simulink model "Sim_Riementrieb"  (Simulink 8.0)
settings: Solver=ode45  StartTime=0.0  StopTime=3.5  MaxStep=1e-3  RelTol=1e-7  AbsTol=1e-7
InitFcn:
  | set_parameter
undefined symbols (not defined in the file or in its folder): mitRegler
libraries: cstblocks x4
settings Model: Creator=wke  LastModifiedBy=cds-lue-1
settings SolverCC: ShapePreserveControl=EnableAll
settings DataIOCC: SignalLoggingSaveFormat=ModelDataLogs
settings DebuggingCC: FcnCallInpInsideContextMsg=UseLocalSettings  StrictBusMsg=Warning
settings SFSimCC: SimParseCustomCode=off
settings CodeAppCC: CustomSymbolStrType=$N$R$M_T  InternalIdentifier=Shortened
settings GRTTargetCC: CombineOutputUpdateFcns=off  GRTInterface=on

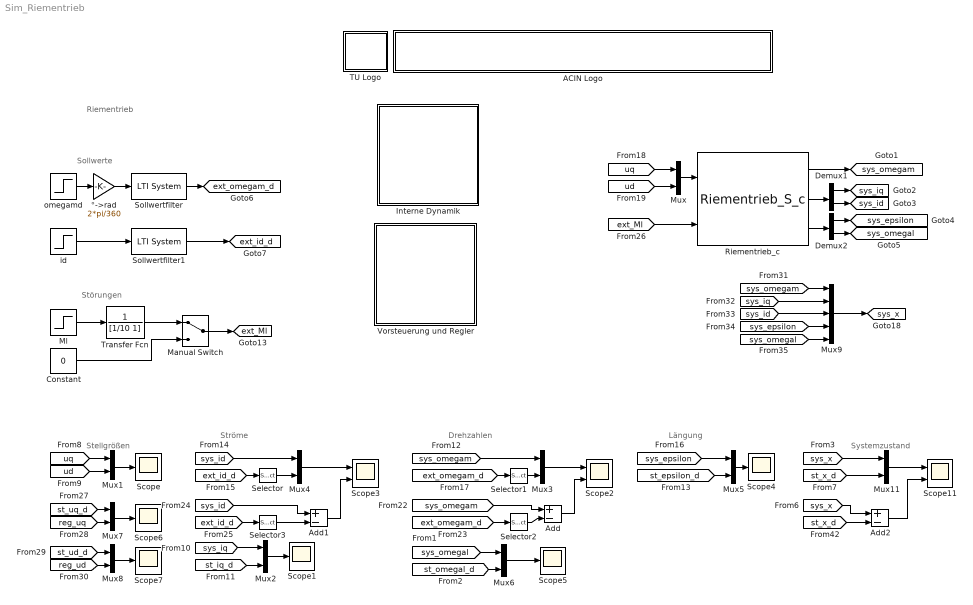
== system Sim_Riementrieb ==
  note: Riementrieb
  note: Sollwerte
  note: Stellgrößen
  note: Ströme
  note: Drehzahlen
  note: Längung
  note: Störungen
  note: Systemzustand
  ACIN Logo : Subsystem
      mask init:
      | s = get_param(gcb,'UserData');
      mask Display:
      | image(s.logo,[0 0 439 45]);
      | %axis image
  Add : Sum  Inputs=+-
  Add1 : Sum  Inputs=+-
  Add2 : Sum  Inputs=+-
  Constant : Constant  Value=0
  Demux1 : Demux  Outputs=2
  Demux2 : Demux  Outputs=2
  Interne Dynamik : Subsystem
  Manual Switch : ManualSwitch
  Ml : Step  Time=2.5  After=0.1  SampleTime=0
  Mux{,1..8,11} (10 alike) : Mux  Inputs=2
  Mux9 : Mux  Inputs=5
  Riementrieb_c : S-Function  FunctionName=Riementrieb_S_c  Parameters=parSys  EnableBusSupport=off
      mask Display:
      | port_label('input',1,'uq,ud');
      | port_label('input',2,'Ml');
      | port_label('output',1,'omegam');
      | port_label('output',2,'iq,id');
      | port_label('output',3,'epsilon,omegal');
  Scope{,1,4..7} (6 alike) : Scope
      Scope settings: YMin=-1  YMax=1
      Scope1 settings: YMin=-300000  YMax=275000
      Scope4 settings: YMin=-0.008  YMax=0.008  SaveName=ScopeData4
      Scope5 settings: YMin=0  YMax=7  SaveName=ScopeData5
      Scope6 settings: YMin=-1.66533e-016  YMax=2.4  SaveName=ScopeData6
      Scope7 settings: YMin=-1.66533e-016  YMax=2.4  SaveName=ScopeData7
  Scope11 : Scope  NumInputPorts=2
      settings: YMin=-300000~-5  YMax=275000~5  SaveName=ScopeData11
  Scope2 : Scope  NumInputPorts=2
      settings: TimeRange=0.3051681706316654  YMin=104.717~-0.0031225  YMax=104.72~-0.00282512  SaveName=ScopeData2
  Scope3 : Scope  NumInputPorts=2
      settings: TimeRange=1.762100082034454  YMin=0.00508121~-5  YMax=0.107262~5  SaveName=ScopeData3
  Selector : Selector  InputPortWidth=2  IndexOptions=Index vector (dialog)  Indices=[1]  OutputSizes=1
  Selector1 : Selector  InputPortWidth=3  IndexOptions=Index vector (dialog)  Indices=[1]  OutputSizes=1
  Selector2 : Selector  InputPortWidth=3  IndexOptions=Index vector (dialog)  Indices=[1]  OutputSizes=1
  Selector3 : Selector  InputPortWidth=2  IndexOptions=Index vector (dialog)  Indices=[1]  OutputSizes=1
  Sollwertfilter : cstblocks/LTI System  sys=parReg.ssSF  IC=[]
  Sollwertfilter1 : cstblocks/LTI System  sys=parReg.ssSFi  IC=[]
  TU Logo : Subsystem
      mask init:
      | s = get_param(gcb,'UserData');
      mask Display: image(s.logo,[0 0 45 45]);
  Transfer Fcn : TransferFcn  Denominator=[1/10 1]
  Vorsteuerung und Regler : Subsystem
  id : Step  Time=0.5  After=0.1  SampleTime=0
  omegamd : Step  Time=1.5  After=1000/60*360  SampleTime=0
  °->rad : Gain  Gain=2*pi/360
  tag scope: ext_Ml=global, ext_id_d=global, ext_omegam_d=global, sys_epsilon=global, sys_id=global, sys_iq=global, sys_omegal=global, sys_omegam=global, sys_x=global
  wires:
  Mux/1 -> Riementrieb_c/1
  °->rad/1 -> Sollwertfilter/1
  Sollwertfilter/1 -> [ext_omegam_d]
  Demux1/1 -> [sys_iq]
  Demux1/2 -> [sys_id]
  Demux2/1 -> [sys_epsilon]
  Demux2/2 -> [sys_omegal]
  Sollwertfilter1/1 -> [ext_id_d]
  id/1 -> Sollwertfilter1/1
  [uq] -> Mux1/1
  [ud] -> Mux1/2
  Mux1/1 -> Scope/1
  [sys_iq] -> Mux2/1
  [st_iq_d] -> Mux2/2
  Mux2/1 -> Scope1/1
  [sys_omegam] -> Mux3/1
  Mux3/1 -> Scope2/1
  [sys_id] -> Mux4/1
  [ext_id_d] -> Selector/1
  Mux4/1 -> Scope3/1
  [sys_epsilon] -> Mux5/1
  Mux5/1 -> Scope4/1
  [sys_omegal] -> Mux6/1
  Mux6/1 -> Scope5/1
  [ext_omegam_d] -> Selector1/1
  Selector1/1 -> Mux3/2
  Selector/1 -> Mux4/2
  [st_epsilon_d] -> Mux5/2
  [st_omegal_d] -> Mux6/2
  Add/1 -> Scope2/2
  [sys_omegam] -> Add/1
  [ext_omegam_d] -> Selector2/1
  Selector2/1 -> Add/2
  Add1/1 -> Scope3/2
  [sys_id] -> Add1/1
  [ext_id_d] -> Selector3/1
  Selector3/1 -> Add1/2
  Ml/1 -> Transfer Fcn/1
  omegamd/1 -> °->rad/1
  [ext_Ml] -> Riementrieb_c/2
  [st_uq_d] -> Mux7/1
  [reg_uq] -> Mux7/2
  Mux7/1 -> Scope6/1
  [st_ud_d] -> Mux8/1
  [reg_ud] -> Mux8/2
  Mux8/1 -> Scope7/1
  Riementrieb_c/2 -> Demux1/1
  Riementrieb_c/3 -> Demux2/1
  Riementrieb_c/1 -> [sys_omegam]
  [sys_omegam] -> Mux9/1
  [sys_iq] -> Mux9/2
  [sys_id] -> Mux9/3
  [sys_epsilon] -> Mux9/4
  [sys_omegal] -> Mux9/5
  Mux9/1 -> [sys_x]
  Mux11/1 -> Scope11/1
  [sys_x] -> Mux11/1
  [st_x_d] -> Mux11/2
  [uq] -> Mux/1
  [ud] -> Mux/2
  Add2/1 -> Scope11/2
  [sys_x] -> Add2/1
  [st_x_d] -> Add2/2
  Transfer Fcn/1 -> Manual Switch/1
  Constant/1 -> Manual Switch/2
  Manual Switch/1 -> [ext_Ml]

== system Sim_Riementrieb/ACIN Logo ==

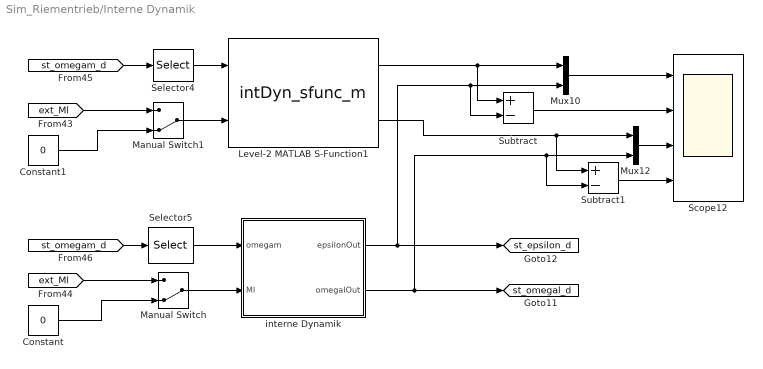
== system Sim_Riementrieb/Interne Dynamik ==
  Constant : Constant  Value=0
  Constant1 : Constant  Value=0
  Level-2 MATLAB S-Function1 : M-S-Function  FunctionName=intDyn_sfunc_m  Parameters=parIndDyn
  Manual Switch : ManualSwitch  CurrentSetting=0
  Manual Switch1 : ManualSwitch  CurrentSetting=0
  Mux10 : Mux  Inputs=2
  Mux12 : Mux  Inputs=2
  Scope12 : Scope  NumInputPorts=4
      settings: YMin=-5~-5~-5~-5  YMax=5~5~5~5  SaveName=ScopeData12
  Selector4 : Selector  InputPortWidth=3  IndexOptions=Index vector (dialog)  Indices=[1]  OutputSizes=1
  Selector5 : Selector  InputPortWidth=3  IndexOptions=Index vector (dialog)  Indices=[1]  OutputSizes=1
  Subtract : Sum  Inputs=+-
  Subtract1 : Sum  Inputs=+-
  interne Dynamik : MATLAB Function  TreatAsAtomicUnit=on
  tag scope: st_epsilon_d=global, st_omegal_d=global
  wires:
  Mux12/1 -> Scope12/3
  Level-2 MATLAB S-Function1/1 -> Mux10/1, Subtract/1
  Subtract1/1 -> Scope12/4
  interne Dynamik/1(epsilonOut) -> Mux10/2, Subtract/2, [st_epsilon_d]
  Subtract/1 -> Scope12/2
  interne Dynamik/2(omegalOut) -> Subtract1/2, Mux12/2, [st_omegal_d]
  [st_omegam_d] -> Selector4/1
  Selector4/1 -> Level-2 MATLAB S-Function1/1
  Level-2 MATLAB S-Function1/2 -> Subtract1/1, Mux12/1
  Mux10/1 -> Scope12/1
  Selector5/1 -> interne Dynamik/1(omegam)
  [st_omegam_d] -> Selector5/1
  Manual Switch/1 -> interne Dynamik/2(Ml)
  [ext_Ml] -> Manual Switch/1
  Constant/1 -> Manual Switch/2
  Manual Switch1/1 -> Level-2 MATLAB S-Function1/2
  [ext_Ml] -> Manual Switch1/1
  Constant1/1 -> Manual Switch1/2

== system Sim_Riementrieb/TU Logo ==

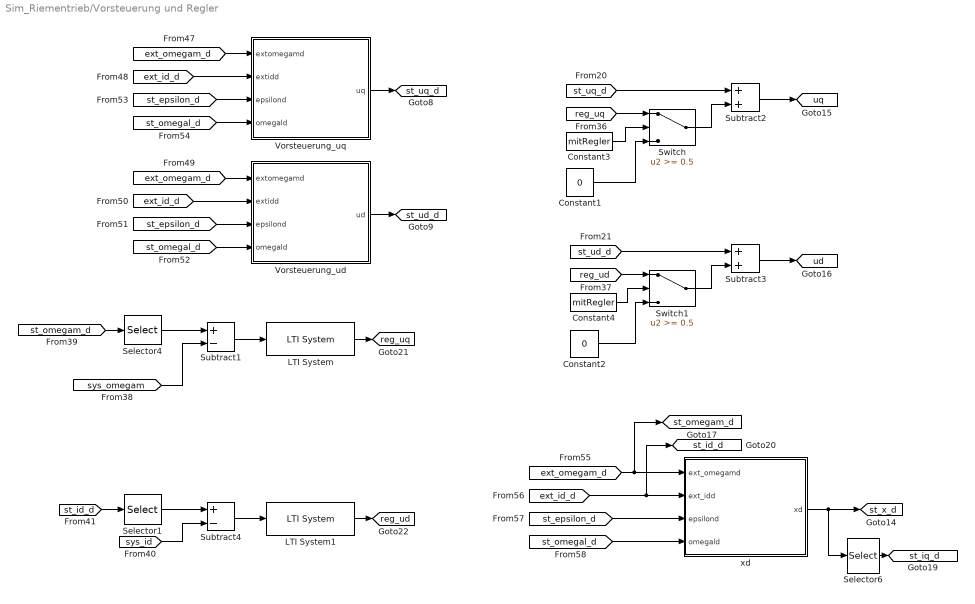
== system Sim_Riementrieb/Vorsteuerung und Regler ==
  Constant1 : Constant  Value=0
  Constant2 : Constant  Value=0
  Constant3 : Constant  Value=mitRegler
  Constant4 : Constant  Value=mitRegler
  LTI System : cstblocks/LTI System  sys=Rz_uq  IC=[]
  LTI System1 : cstblocks/LTI System  sys=Rz_ud  IC=[]
  Selector1 : Selector  InputPortWidth=2  IndexOptions=Index vector (dialog)  Indices=[1]  OutputSizes=1
  Selector4 : Selector  InputPortWidth=3  IndexOptions=Index vector (dialog)  Indices=[1]  OutputSizes=1
  Selector6 : Selector  InputPortWidth=5  IndexOptions=Index vector (dialog)  Indices=[2]  OutputSizes=1
  Subtract1 : Sum  Inputs=+-
  Subtract2 : Sum
  Subtract3 : Sum
  Subtract4 : Sum  Inputs=+-
  Switch : Switch  Threshold=0.5
  Switch1 : Switch  Threshold=0.5
  Vorsteuerung_ud : MATLAB Function  TreatAsAtomicUnit=on
  Vorsteuerung_uq : MATLAB Function  TreatAsAtomicUnit=on
  xd : MATLAB Function  TreatAsAtomicUnit=on
  tag scope: reg_ud=global, reg_uq=global, st_id_d=global, st_iq_d=global, st_omegam_d=global, st_ud_d=global, st_uq_d=global, st_x_d=global, ud=global, uq=global
  wires:
  [st_uq_d] -> Subtract2/1
  Constant2/1 -> Switch1/3
  Constant3/1 -> Switch/2
  Constant4/1 -> Switch1/2
  Switch1/1 -> Subtract3/2
  [st_ud_d] -> Subtract3/1
  Constant1/1 -> Switch/3
  Subtract3/1 -> [ud]
  [ext_id_d] -> [st_id_d], xd/2(ext_idd)
  [ext_omegam_d] -> [st_omegam_d], xd/1(ext_omegamd)
  [st_omegal_d] -> xd/4(omegald)
  [st_epsilon_d] -> xd/3(epsilond)
  [reg_uq] -> Switch/1
  Switch/1 -> Subtract2/2
  xd/1(xd) -> Selector6/1, [st_x_d]
  [reg_ud] -> Switch1/1
  [st_epsilon_d] -> Vorsteuerung_uq/3(epsilond)
  [st_omegal_d] -> Vorsteuerung_uq/4(omegald)
  Vorsteuerung_uq/1(uq) -> [st_uq_d]
  Vorsteuerung_ud/1(ud) -> [st_ud_d]
  [st_epsilon_d] -> Vorsteuerung_ud/3(epsilond)
  [ext_id_d] -> Vorsteuerung_ud/2(extidd)
  [ext_omegam_d] -> Vorsteuerung_ud/1(extomegamd)
  [ext_id_d] -> Vorsteuerung_uq/2(extidd)
  [ext_omegam_d] -> Vorsteuerung_uq/1(extomegamd)
  [st_omegal_d] -> Vorsteuerung_ud/4(omegald)
  Selector6/1 -> [st_iq_d]
  Subtract2/1 -> [uq]
  LTI System/1 -> [reg_uq]
  LTI System1/1 -> [reg_ud]
  Subtract1/1 -> LTI System/1
  Subtract4/1 -> LTI System1/1
  [st_omegam_d] -> Selector4/1
  Selector4/1 -> Subtract1/1
  [sys_omegam] -> Subtract1/2
  Selector1/1 -> Subtract4/1
  [st_id_d] -> Selector1/1
  [sys_id] -> Subtract4/2

== matlab function Vorsteuerung und Regler/Vorsteuerung_uq ==
  settings: updateMethod=DISCRETE  sampleTime=parSys.Ta
  data: extomegamd input double; extidd input double; epsilond input double; omegald input double; uq output double; parSys parameter double
function uq = Vorsteuerung_uq(extomegamd, extidd, epsilond, omegald ,parSys)

omegamd = extomegamd(1);
omegamdp = extomegamd(2);
omegamd2p = extomegamd(3);

idd = extidd(1);
iddp = extidd(2);


Il = parSys.Il;
cr1 = parSys.cr1;
cr3 = parSys.cr3;
dl = parSys.dl;
rl = parSys.rl;
Imot = parSys.Im;
dm = parSys.dm;
rm = parSys.rm;
Rm = parSys.Rm;
Lm = parSys.Lm;
p = parSys.p;
Phi = parSys.Phi;



iqd = 0.2e1 / 0.3e1 * (-2 * cr3 * rm * epsilond ^ 3 - 2 * cr1 * rm * epsilond + Imot * omegamdp + dm * omegamd) / Phi / p;


uq = Lm * Imot / Phi / p * (omegamd2p + 0.1e1 / Imot ^ 2 * dm * ((2 * (cr3 * epsilond ^ 3 + cr1 * epsilond) * rm) - dm * omegamd + 0.3e1 / 0.2e1 * p * Phi * iqd) - 0.1e1 / Imot * Phi * p * (0.3e1 * Lm * idd * omegamd * p - 0.2e1 * Phi * omegamd * p - 0.2e1 * Rm * iqd) / Lm / 0.2e1 - 0.2e1 / Imot * (3 * cr3 * epsilond ^ 2 + cr1) * rm * (omegald * rl - omegamd * rm));


end

== matlab function Interne Dynamik/interne Dynamik ==
  settings: updateMethod=DISCRETE  sampleTime=parSys.TsID
  data: omegam input double; epsilonOut output double; Ml input double; omegalOut output double; parSys parameter double
function [epsilonOut, omegalOut] = intDyn(omegam, Ml, parSys)

persistent epsilon;
persistent omegal;
persistent epsilonAlt;
persistent omegalAlt;
persistent omegamAlt;
persistent MlAlt;

if isempty(epsilon)
    epsilon  = parSys.eta_1_0;
end
if isempty(omegal)
    omegal = parSys.eta_2_0;
end
if isempty(epsilonAlt)
    epsilonAlt  = parSys.eta_1_0;
end
if isempty(omegalAlt)
    omegalAlt = parSys.eta_2_0;
end

if isempty(omegamAlt)
    omegamAlt = 0;
end
if isempty(MlAlt)
    MlAlt = 0;
end

% Parameter einlesen
cr1 = parSys.cr1;
cr3 = parSys.cr3;
rl = parSys.rl;
rm = parSys.rm;
Il = parSys.Il;
dl = parSys.dl;
TsID = parSys.TsID;


% Riemenkraft
FrAlt = cr3 * epsilonAlt ^ 3 + cr1 * epsilonAlt;

% Heun Algorithmus für epsilon
    % Vorhersagungsschritt
    epsilonP = epsilonAlt + TsID*(omegalAlt*rl - omegamAlt*rm);
    omegalP = omegalAlt + TsID * 1/Il * (-2*FrAlt*rl - dl*omegamAlt + MlAlt);

    % Verbesserungsschritt
    FrNeu = cr3 * epsilonP ^ 3 + cr1 * epsilonP;
    epsilonNeu = epsilonAlt + TsID/2 * ((omegalAlt*rl - omegamAlt*rm) + (omegalP*rl - omegam*rm));
    omegalNeu = omegalAlt +  TsID/2 * (1/Il * (-2*FrAlt*rl - dl*omegalAlt + MlAlt) + 1/Il * (-2*FrNeu*rl - dl*omegalP + Ml));

% Ausgabe
epsilonOut = epsilonNeu;
omegalOut = omegalNeu;

% Merken für erneuten Berechnungsschritt
epsilonAlt = epsilonNeu;
omegalAlt = omegalNeu;

MlAlt = Ml;
omegamAlt = omegam;


end

== matlab function Vorsteuerung und Regler/Vorsteuerung_ud ==
  settings: updateMethod=DISCRETE  sampleTime=parSys.Ta
  data: extomegamd input double; extidd input double; epsilond input double; omegald input double; ud output double; parSys parameter double
function ud = Vorsteuerung_ud(extomegamd, extidd, epsilond, omegald ,parSys)

omegamd = extomegamd(1);
omegamdp = extomegamd(2);
omegamd2p = extomegamd(3);

idd = extidd(1);
iddp = extidd(2);


Il = parSys.Il;
cr1 = parSys.cr1;
cr3 = parSys.cr3;
dl = parSys.dl;
rl = parSys.rl;
Imot = parSys.Im;
dm = parSys.dm;
rm = parSys.rm;
Rm = parSys.Rm;
Lm = parSys.Lm;
p = parSys.p;
Phi = parSys.Phi;



iqd = 0.2e1 / 0.3e1 * (-2 * cr3 * rm * epsilond ^ 3 - 2 * cr1 * rm * epsilond + Imot * omegamdp + dm * omegamd) / Phi / p;

ud = 0.3e1 / 0.2e1 * Lm * (iddp + ((3 * Lm * iqd * omegamd * p + 2 * Rm * idd) / Lm) / 0.3e1);

end

== matlab function Vorsteuerung und Regler/xd ==
  settings: updateMethod=DISCRETE  sampleTime=parSys.Ta
  data: ext_omegamd input double; ext_idd input double; epsilond input double; omegald input double; xd output double; parSys parameter double
function xd = xd(ext_omegamd, ext_idd, epsilond, omegald, parSys)

omegamd = ext_omegamd(1);
omegamdp = ext_omegamd(2);

idd = ext_idd(1);

Il = parSys.Il;
cr1 = parSys.cr1;
cr3 = parSys.cr3;
dl = parSys.dl;
rl = parSys.rl;
Imot = parSys.Im;
dm = parSys.dm;
rm = parSys.rm;
Rm = parSys.Rm;
Lm = parSys.Lm;
p = parSys.p;
Phi = parSys.Phi;


xd = [omegamd 0.2e1 / 0.3e1 * (-2 * cr3 * rm * epsilond ^ 3 - 2 * cr1 * rm * epsilond + Imot * omegamdp + dm * omegamd) / Phi / p idd epsilond omegald];


end
